simulink model "dec_2"  (R2013b)
settings: Solver=ode45  StartTime=0.0  StopTime=2500  RelTol=1e-3
undefined symbols (not defined in the file or in its folder): pfb_coeff_gen_calc, xlfda_numerator, xlipgetpartsetting
libraries: xbsIndex_r4 x1575, casper_library_delays x21, dspsigops x16, casper_library_misc x9, simulink x1, xps_library x1
(part 5 of 15)

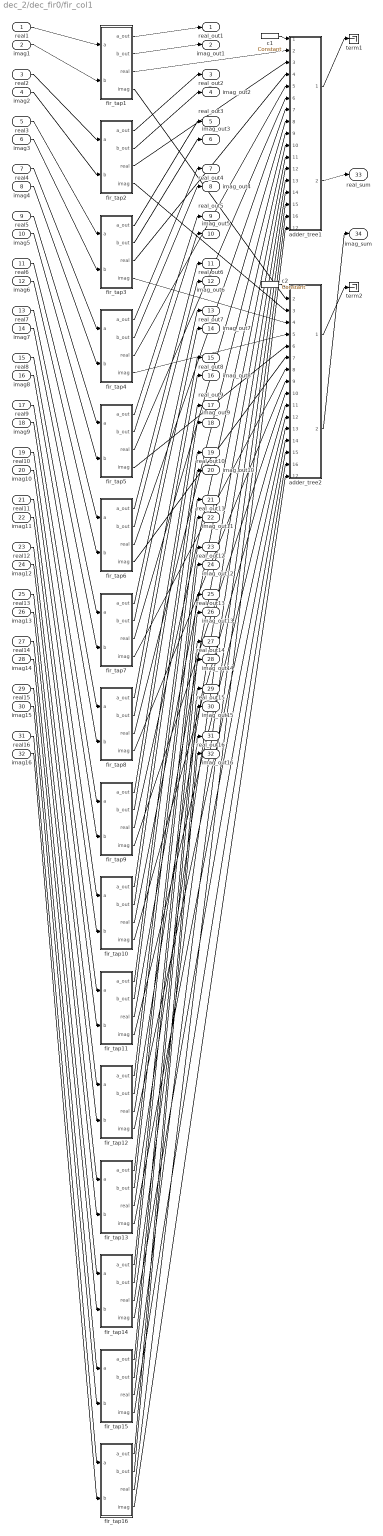
== system dec_2/dec_fir0/fir_col1 ==
  real1 : Inport
  imag1 : Inport  Port=2
  real2 : Inport  Port=3
  imag2 : Inport  Port=4
  real3 : Inport  Port=5
  imag3 : Inport  Port=6
  real4 : Inport  Port=7
  imag4 : Inport  Port=8
  real5 : Inport  Port=9
  imag5 : Inport  Port=10
  real6 : Inport  Port=11
  imag6 : Inport  Port=12
  real7 : Inport  Port=13
  imag7 : Inport  Port=14
  real8 : Inport  Port=15
  imag8 : Inport  Port=16
  real9 : Inport  Port=17
  imag9 : Inport  Port=18
  real10 : Inport  Port=19
  imag10 : Inport  Port=20
  real11 : Inport  Port=21
  imag11 : Inport  Port=22
  real12 : Inport  Port=23
  imag12 : Inport  Port=24
  real13 : Inport  Port=25
  imag13 : Inport  Port=26
  real14 : Inport  Port=27
  imag14 : Inport  Port=28
  real15 : Inport  Port=29
  imag15 : Inport  Port=30
  real16 : Inport  Port=31
  imag16 : Inport  Port=32
  adder_tree1 : Subsystem  AncestorBlock=casper_library_misc/adder_tree  mask(adder_tree){n_inputs=16, latency=1, adder_imp=DSP48, first_stage_hdl=on}
      mask prompts: n_inputs "Number of Inputs"; latency "Add Latency"; adder_imp "Adder implementation"; first_stage_hdl "Use behavioural HDL for first stage of adders"
      mask help:
      | Sums all inputs using a tree of adds and delays.
      |
      | Number of inputs: The number of inputs to the block to be summed
      | Add latency: The number of clock cycles to perform one addition (affects timing)..
      | Adder implementation: choice of fabric or DSP48E core, or behavioral HDL
      | Use behavioural HDL for first stage of adders: Causes the first stage of adders to be absorbed into DSP blocks if multipliers precede them (Virtex 5). Overrides Adder implementation
      mask init:
      | adder_tree_init(gcb, ...
      |     'n_inputs', n_inputs, ...
      |     'latency', latency, ...
      |     'adder_imp', adder_imp, ...
      |     'first_stage_hdl', first_stage_hdl);
      settings: AttributesFormatString=latency 4
      mask Help: eval('xlWeb(''http://casper.berkeley.edu/wiki/Adder_tree'')')
      mask TypeOptions adder_imp: Behavioral | Fabric | DSP48
  adder_tree2 : Subsystem  AncestorBlock=casper_library_misc/adder_tree  mask(adder_tree){n_inputs=16, latency=1, adder_imp=DSP48, first_stage_hdl=on}
      mask prompts: n_inputs "Number of Inputs"; latency "Add Latency"; adder_imp "Adder implementation"; first_stage_hdl "Use behavioural HDL for first stage of adders"
      mask help:
      | Sums all inputs using a tree of adds and delays.
      |
      | Number of inputs: The number of inputs to the block to be summed
      | Add latency: The number of clock cycles to perform one addition (affects timing)..
      | Adder implementation: choice of fabric or DSP48E core, or behavioral HDL
      | Use behavioural HDL for first stage of adders: Causes the first stage of adders to be absorbed into DSP blocks if multipliers precede them (Virtex 5). Overrides Adder implementation
      mask init:
      | adder_tree_init(gcb, ...
      |     'n_inputs', n_inputs, ...
      |     'latency', latency, ...
      |     'adder_imp', adder_imp, ...
      |     'first_stage_hdl', first_stage_hdl);
      settings: AttributesFormatString=latency 4
      mask Help: eval('xlWeb(''http://casper.berkeley.edu/wiki/Adder_tree'')')
      mask TypeOptions adder_imp: Behavioral | Fabric | DSP48
  c1 : xbsIndex_r4/Constant  const=1  gui_display_data_type=Fixed-point  arith_type=Signed (2's comp)  n_bits=16  bin_pt=14  preci_type=Single  exp_width=8  frac_width=24  explicit_period=on  period=1  equ=P=C  opselect=C  inp2=PCIN>>17  opr=+  inp1=P  carry=CIN  dbl_ovrd=off  block_type=constant
  c2 : xbsIndex_r4/Constant  const=1  gui_display_data_type=Fixed-point  arith_type=Signed (2's comp)  n_bits=16  bin_pt=14  preci_type=Single  exp_width=8  frac_width=24  explicit_period=on  period=1  equ=P=C  opselect=C  inp2=PCIN>>17  opr=+  inp1=P  carry=CIN  dbl_ovrd=off  block_type=constant
  fir_tap1 : Subsystem  AncestorBlock=casper_library_downconverter/fir_tap  mask(fir_tap){factor=0.0062127, latency=2, coeff_bit_width=25, coeff_bin_pt=24}
      mask prompts: latency "Mult latency"; coeff_bit_width "Coefficient bit width"; coeff_bin_pt "Coefficient binary point"
      mask help: Multiplies input data with factor specified.
      mask init:
      | fir_tap_init(gcb, ...
      |     'factor', factor, ...
      |     'latency', latency, ...
      |     'coeff_bit_width', coeff_bit_width, ...
      |     'coeff_bin_pt', coeff_bin_pt);
      mask Help: eval('xlWeb(''http://casper.berkeley.edu/wiki/Fir_tap'')')
  fir_tap10 : Subsystem  AncestorBlock=casper_library_downconverter/fir_tap  mask(fir_tap){factor=-0.0033818, latency=2, coeff_bit_width=25, coeff_bin_pt=24}
      mask prompts: latency "Mult latency"; coeff_bit_width "Coefficient bit width"; coeff_bin_pt "Coefficient binary point"
      mask help: Multiplies input data with factor specified.
      mask init:
      | fir_tap_init(gcb, ...
      |     'factor', factor, ...
      |     'latency', latency, ...
      |     'coeff_bit_width', coeff_bit_width, ...
      |     'coeff_bin_pt', coeff_bin_pt);
      mask Help: eval('xlWeb(''http://casper.berkeley.edu/wiki/Fir_tap'')')
  fir_tap11 : Subsystem  AncestorBlock=casper_library_downconverter/fir_tap  mask(fir_tap){factor=-0.0039996, latency=2, coeff_bit_width=25, coeff_bin_pt=24}
      mask prompts: latency "Mult latency"; coeff_bit_width "Coefficient bit width"; coeff_bin_pt "Coefficient binary point"
      mask help: Multiplies input data with factor specified.
      mask init:
      | fir_tap_init(gcb, ...
      |     'factor', factor, ...
      |     'latency', latency, ...
      |     'coeff_bit_width', coeff_bit_width, ...
      |     'coeff_bin_pt', coeff_bin_pt);
      mask Help: eval('xlWeb(''http://casper.berkeley.edu/wiki/Fir_tap'')')
  fir_tap12 : Subsystem  AncestorBlock=casper_library_downconverter/fir_tap  mask(fir_tap){factor=-0.0044174, latency=2, coeff_bit_width=25, coeff_bin_pt=24}
      mask prompts: latency "Mult latency"; coeff_bit_width "Coefficient bit width"; coeff_bin_pt "Coefficient binary point"
      mask help: Multiplies input data with factor specified.
      mask init:
      | fir_tap_init(gcb, ...
      |     'factor', factor, ...
      |     'latency', latency, ...
      |     'coeff_bit_width', coeff_bit_width, ...
      |     'coeff_bin_pt', coeff_bin_pt);
      mask Help: eval('xlWeb(''http://casper.berkeley.edu/wiki/Fir_tap'')')
  fir_tap13 : Subsystem  AncestorBlock=casper_library_downconverter/fir_tap  mask(fir_tap){factor=-0.0046295, latency=2, coeff_bit_width=25, coeff_bin_pt=24}
      mask prompts: latency "Mult latency"; coeff_bit_width "Coefficient bit width"; coeff_bin_pt "Coefficient binary point"
      mask help: Multiplies input data with factor specified.
      mask init:
      | fir_tap_init(gcb, ...
      |     'factor', factor, ...
      |     'latency', latency, ...
      |     'coeff_bit_width', coeff_bit_width, ...
      |     'coeff_bin_pt', coeff_bin_pt);
      mask Help: eval('xlWeb(''http://casper.berkeley.edu/wiki/Fir_tap'')')
  fir_tap14 : Subsystem  AncestorBlock=casper_library_downconverter/fir_tap  mask(fir_tap){factor=-0.0046386, latency=2, coeff_bit_width=25, coeff_bin_pt=24}
      mask prompts: latency "Mult latency"; coeff_bit_width "Coefficient bit width"; coeff_bin_pt "Coefficient binary point"
      mask help: Multiplies input data with factor specified.
      mask init:
      | fir_tap_init(gcb, ...
      |     'factor', factor, ...
      |     'latency', latency, ...
      |     'coeff_bit_width', coeff_bit_width, ...
      |     'coeff_bin_pt', coeff_bin_pt);
      mask Help: eval('xlWeb(''http://casper.berkeley.edu/wiki/Fir_tap'')')
  fir_tap15 : Subsystem  AncestorBlock=casper_library_downconverter/fir_tap  mask(fir_tap){factor=-0.0044554, latency=2, coeff_bit_width=25, coeff_bin_pt=24}
      mask prompts: latency "Mult latency"; coeff_bit_width "Coefficient bit width"; coeff_bin_pt "Coefficient binary point"
      mask help: Multiplies input data with factor specified.
      mask init:
      | fir_tap_init(gcb, ...
      |     'factor', factor, ...
      |     'latency', latency, ...
      |     'coeff_bit_width', coeff_bit_width, ...
      |     'coeff_bin_pt', coeff_bin_pt);
      mask Help: eval('xlWeb(''http://casper.berkeley.edu/wiki/Fir_tap'')')
  fir_tap16 : Subsystem  AncestorBlock=casper_library_downconverter/fir_tap  mask(fir_tap){factor=-0.0040983, latency=2, coeff_bit_width=25, coeff_bin_pt=24}
      mask prompts: latency "Mult latency"; coeff_bit_width "Coefficient bit width"; coeff_bin_pt "Coefficient binary point"
      mask help: Multiplies input data with factor specified.
      mask init:
      | fir_tap_init(gcb, ...
      |     'factor', factor, ...
      |     'latency', latency, ...
      |     'coeff_bit_width', coeff_bit_width, ...
      |     'coeff_bin_pt', coeff_bin_pt);
      mask Help: eval('xlWeb(''http://casper.berkeley.edu/wiki/Fir_tap'')')
  fir_tap2 : Subsystem  AncestorBlock=casper_library_downconverter/fir_tap  mask(fir_tap){factor=0.0053266, latency=2, coeff_bit_width=25, coeff_bin_pt=24}
      mask prompts: latency "Mult latency"; coeff_bit_width "Coefficient bit width"; coeff_bin_pt "Coefficient binary point"
      mask help: Multiplies input data with factor specified.
      mask init:
      | fir_tap_init(gcb, ...
      |     'factor', factor, ...
      |     'latency', latency, ...
      |     'coeff_bit_width', coeff_bit_width, ...
      |     'coeff_bin_pt', coeff_bin_pt);
      mask Help: eval('xlWeb(''http://casper.berkeley.edu/wiki/Fir_tap'')')
  fir_tap3 : Subsystem  AncestorBlock=casper_library_downconverter/fir_tap  mask(fir_tap){factor=0.0042757, latency=2, coeff_bit_width=25, coeff_bin_pt=24}
      mask prompts: latency "Mult latency"; coeff_bit_width "Coefficient bit width"; coeff_bin_pt "Coefficient binary point"
      mask help: Multiplies input data with factor specified.
      mask init:
      | fir_tap_init(gcb, ...
      |     'factor', factor, ...
      |     'latency', latency, ...
      |     'coeff_bit_width', coeff_bit_width, ...
      |     'coeff_bin_pt', coeff_bin_pt);
      mask Help: eval('xlWeb(''http://casper.berkeley.edu/wiki/Fir_tap'')')
  fir_tap4 : Subsystem  AncestorBlock=casper_library_downconverter/fir_tap  mask(fir_tap){factor=0.0031122, latency=2, coeff_bit_width=25, coeff_bin_pt=24}
      mask prompts: latency "Mult latency"; coeff_bit_width "Coefficient bit width"; coeff_bin_pt "Coefficient binary point"
      mask help: Multiplies input data with factor specified.
      mask init:
      | fir_tap_init(gcb, ...
      |     'factor', factor, ...
      |     'latency', latency, ...
      |     'coeff_bit_width', coeff_bit_width, ...
      |     'coeff_bin_pt', coeff_bin_pt);
      mask Help: eval('xlWeb(''http://casper.berkeley.edu/wiki/Fir_tap'')')
  fir_tap5 : Subsystem  AncestorBlock=casper_library_downconverter/fir_tap  mask(fir_tap){factor=0.00189, latency=2, coeff_bit_width=25, coeff_bin_pt=24}
      mask prompts: latency "Mult latency"; coeff_bit_width "Coefficient bit width"; coeff_bin_pt "Coefficient binary point"
      mask help: Multiplies input data with factor specified.
      mask init:
      | fir_tap_init(gcb, ...
      |     'factor', factor, ...
      |     'latency', latency, ...
      |     'coeff_bit_width', coeff_bit_width, ...
      |     'coeff_bin_pt', coeff_bin_pt);
      mask Help: eval('xlWeb(''http://casper.berkeley.edu/wiki/Fir_tap'')')
  fir_tap6 : Subsystem  AncestorBlock=casper_library_downconverter/fir_tap  mask(fir_tap){factor=0.00066203, latency=2, coeff_bit_width=25, coeff_bin_pt=24}
      mask prompts: latency "Mult latency"; coeff_bit_width "Coefficient bit width"; coeff_bin_pt "Coefficient binary point"
      mask help: Multiplies input data with factor specified.
      mask init:
      | fir_tap_init(gcb, ...
      |     'factor', factor, ...
      |     'latency', latency, ...
      |     'coeff_bit_width', coeff_bit_width, ...
      |     'coeff_bin_pt', coeff_bin_pt);
      mask Help: eval('xlWeb(''http://casper.berkeley.edu/wiki/Fir_tap'')')
  fir_tap7 : Subsystem  AncestorBlock=casper_library_downconverter/fir_tap  mask(fir_tap){factor=-0.00052147, latency=2, coeff_bit_width=25, coeff_bin_pt=24}
      mask prompts: latency "Mult latency"; coeff_bit_width "Coefficient bit width"; coeff_bin_pt "Coefficient binary point"
      mask help: Multiplies input data with factor specified.
      mask init:
      | fir_tap_init(gcb, ...
      |     'factor', factor, ...
      |     'latency', latency, ...
      |     'coeff_bit_width', coeff_bit_width, ...
      |     'coeff_bin_pt', coeff_bin_pt);
      mask Help: eval('xlWeb(''http://casper.berkeley.edu/wiki/Fir_tap'')')
  fir_tap8 : Subsystem  AncestorBlock=casper_library_downconverter/fir_tap  mask(fir_tap){factor=-0.001615, latency=2, coeff_bit_width=25, coeff_bin_pt=24}
      mask prompts: latency "Mult latency"; coeff_bit_width "Coefficient bit width"; coeff_bin_pt "Coefficient binary point"
      mask help: Multiplies input data with factor specified.
      mask init:
      | fir_tap_init(gcb, ...
      |     'factor', factor, ...
      |     'latency', latency, ...
      |     'coeff_bit_width', coeff_bit_width, ...
      |     'coeff_bin_pt', coeff_bin_pt);
      mask Help: eval('xlWeb(''http://casper.berkeley.edu/wiki/Fir_tap'')')
  fir_tap9 : Subsystem  AncestorBlock=casper_library_downconverter/fir_tap  mask(fir_tap){factor=-0.0025791, latency=2, coeff_bit_width=25, coeff_bin_pt=24}
      mask prompts: latency "Mult latency"; coeff_bit_width "Coefficient bit width"; coeff_bin_pt "Coefficient binary point"
      mask help: Multiplies input data with factor specified.
      mask init:
      | fir_tap_init(gcb, ...
      |     'factor', factor, ...
      |     'latency', latency, ...
      |     'coeff_bit_width', coeff_bit_width, ...
      |     'coeff_bin_pt', coeff_bin_pt);
      mask Help: eval('xlWeb(''http://casper.berkeley.edu/wiki/Fir_tap'')')
  term1 : Terminator
  term2 : Terminator
  real_out1 : Outport
  imag_out1 : Outport  Port=2
  real_out2 : Outport  Port=3
  imag_out2 : Outport  Port=4
  real_out3 : Outport  Port=5
  imag_out3 : Outport  Port=6
  real_out4 : Outport  Port=7
  imag_out4 : Outport  Port=8
  real_out5 : Outport  Port=9
  imag_out5 : Outport  Port=10
  real_out6 : Outport  Port=11
  imag_out6 : Outport  Port=12
  real_out7 : Outport  Port=13
  imag_out7 : Outport  Port=14
  real_out8 : Outport  Port=15
  imag_out8 : Outport  Port=16
  real_out9 : Outport  Port=17
  imag_out9 : Outport  Port=18
  real_out10 : Outport  Port=19
  imag_out10 : Outport  Port=20
  real_out11 : Outport  Port=21
  imag_out11 : Outport  Port=22
  real_out12 : Outport  Port=23
  imag_out12 : Outport  Port=24
  real_out13 : Outport  Port=25
  imag_out13 : Outport  Port=26
  real_out14 : Outport  Port=27
  imag_out14 : Outport  Port=28
  real_out15 : Outport  Port=29
  imag_out15 : Outport  Port=30
  real_out16 : Outport  Port=31
  imag_out16 : Outport  Port=32
  real_sum : Outport  Port=33
  imag_sum : Outport  Port=34
  wires:
  adder_tree1/1(sync_out) -> term1/1
  adder_tree2/1(sync_out) -> term2/1
  c1/1 -> adder_tree1/1(sync)
  c2/1 -> adder_tree2/1(sync)
  adder_tree1/2(dout) -> real_sum/1
  adder_tree2/2(dout) -> imag_sum/1
  real1/1 -> fir_tap1/1(a)
  imag1/1 -> fir_tap1/2(b)
  fir_tap1/1(a_out) -> real_out1/1
  fir_tap1/2(b_out) -> imag_out1/1
  fir_tap1/3(real) -> adder_tree1/2(din1)
  fir_tap1/4(imag) -> adder_tree2/2(din1)
  real2/1 -> fir_tap2/1(a)
  imag2/1 -> fir_tap2/2(b)
  fir_tap2/1(a_out) -> real_out2/1
  fir_tap2/2(b_out) -> imag_out2/1
  fir_tap2/3(real) -> adder_tree1/3(din2)
  fir_tap2/4(imag) -> adder_tree2/3(din2)
  real3/1 -> fir_tap3/1(a)
  imag3/1 -> fir_tap3/2(b)
  fir_tap3/1(a_out) -> real_out3/1
  fir_tap3/2(b_out) -> imag_out3/1
  fir_tap3/3(real) -> adder_tree1/4(din3)
  fir_tap3/4(imag) -> adder_tree2/4(din3)
  real4/1 -> fir_tap4/1(a)
  imag4/1 -> fir_tap4/2(b)
  fir_tap4/1(a_out) -> real_out4/1
  fir_tap4/2(b_out) -> imag_out4/1
  fir_tap4/3(real) -> adder_tree1/5(din4)
  fir_tap4/4(imag) -> adder_tree2/5(din4)
  real5/1 -> fir_tap5/1(a)
  imag5/1 -> fir_tap5/2(b)
  fir_tap5/1(a_out) -> real_out5/1
  fir_tap5/2(b_out) -> imag_out5/1
  fir_tap5/3(real) -> adder_tree1/6(din5)
  fir_tap5/4(imag) -> adder_tree2/6(din5)
  real6/1 -> fir_tap6/1(a)
  imag6/1 -> fir_tap6/2(b)
  fir_tap6/1(a_out) -> real_out6/1
  fir_tap6/2(b_out) -> imag_out6/1
  fir_tap6/3(real) -> adder_tree1/7(din6)
  fir_tap6/4(imag) -> adder_tree2/7(din6)
  real7/1 -> fir_tap7/1(a)
  imag7/1 -> fir_tap7/2(b)
  fir_tap7/1(a_out) -> real_out7/1
  fir_tap7/2(b_out) -> imag_out7/1
  fir_tap7/3(real) -> adder_tree1/8(din7)
  fir_tap7/4(imag) -> adder_tree2/8(din7)
  real8/1 -> fir_tap8/1(a)
  imag8/1 -> fir_tap8/2(b)
  fir_tap8/1(a_out) -> real_out8/1
  fir_tap8/2(b_out) -> imag_out8/1
  fir_tap8/3(real) -> adder_tree1/9(din8)
  fir_tap8/4(imag) -> adder_tree2/9(din8)
  real9/1 -> fir_tap9/1(a)
  imag9/1 -> fir_tap9/2(b)
  fir_tap9/1(a_out) -> real_out9/1
  fir_tap9/2(b_out) -> imag_out9/1
  fir_tap9/3(real) -> adder_tree1/10(din9)
  fir_tap9/4(imag) -> adder_tree2/10(din9)
  real10/1 -> fir_tap10/1(a)
  imag10/1 -> fir_tap10/2(b)
  fir_tap10/1(a_out) -> real_out10/1
  fir_tap10/2(b_out) -> imag_out10/1
  fir_tap10/3(real) -> adder_tree1/11(din10)
  fir_tap10/4(imag) -> adder_tree2/11(din10)
  real11/1 -> fir_tap11/1(a)
  imag11/1 -> fir_tap11/2(b)
  fir_tap11/1(a_out) -> real_out11/1
  fir_tap11/2(b_out) -> imag_out11/1
  fir_tap11/3(real) -> adder_tree1/12(din11)
  fir_tap11/4(imag) -> adder_tree2/12(din11)
  real12/1 -> fir_tap12/1(a)
  imag12/1 -> fir_tap12/2(b)
  fir_tap12/1(a_out) -> real_out12/1
  fir_tap12/2(b_out) -> imag_out12/1
  fir_tap12/3(real) -> adder_tree1/13(din12)
  fir_tap12/4(imag) -> adder_tree2/13(din12)
  real13/1 -> fir_tap13/1(a)
  imag13/1 -> fir_tap13/2(b)
  fir_tap13/1(a_out) -> real_out13/1
  fir_tap13/2(b_out) -> imag_out13/1
  fir_tap13/3(real) -> adder_tree1/14(din13)
  fir_tap13/4(imag) -> adder_tree2/14(din13)
  real14/1 -> fir_tap14/1(a)
  imag14/1 -> fir_tap14/2(b)
  fir_tap14/1(a_out) -> real_out14/1
  fir_tap14/2(b_out) -> imag_out14/1
  fir_tap14/3(real) -> adder_tree1/15(din14)
  fir_tap14/4(imag) -> adder_tree2/15(din14)
  real15/1 -> fir_tap15/1(a)
  imag15/1 -> fir_tap15/2(b)
  fir_tap15/1(a_out) -> real_out15/1
  fir_tap15/2(b_out) -> imag_out15/1
  fir_tap15/3(real) -> adder_tree1/16(din15)
  fir_tap15/4(imag) -> adder_tree2/16(din15)
  real16/1 -> fir_tap16/1(a)
  imag16/1 -> fir_tap16/2(b)
  fir_tap16/1(a_out) -> real_out16/1
  fir_tap16/2(b_out) -> imag_out16/1
  fir_tap16/3(real) -> adder_tree1/17(din16)
  fir_tap16/4(imag) -> adder_tree2/17(din16)

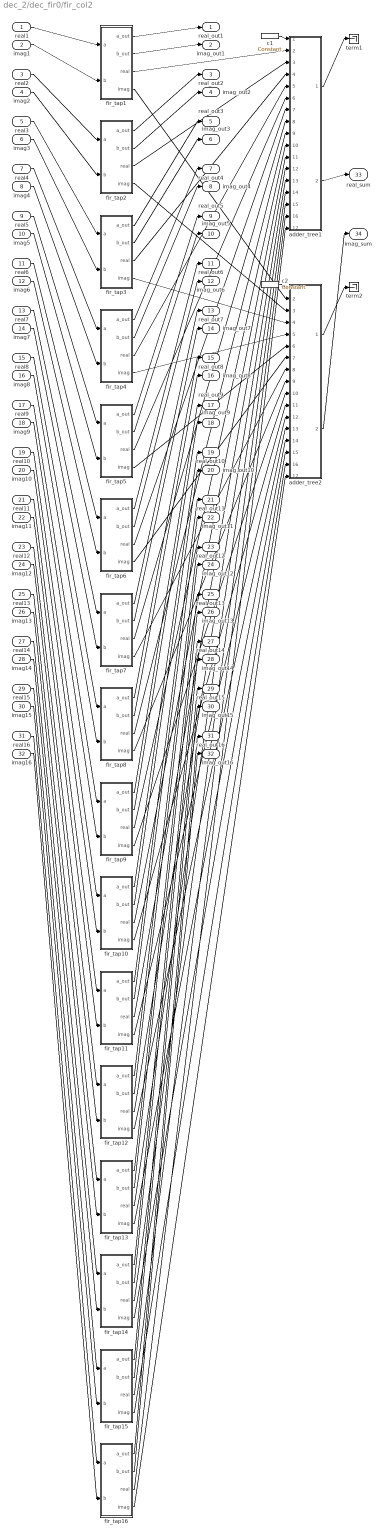
== system dec_2/dec_fir0/fir_col2 ==
  real1 : Inport
  imag1 : Inport  Port=2
  real2 : Inport  Port=3
  imag2 : Inport  Port=4
  real3 : Inport  Port=5
  imag3 : Inport  Port=6
  real4 : Inport  Port=7
  imag4 : Inport  Port=8
  real5 : Inport  Port=9
  imag5 : Inport  Port=10
  real6 : Inport  Port=11
  imag6 : Inport  Port=12
  real7 : Inport  Port=13
  imag7 : Inport  Port=14
  real8 : Inport  Port=15
  imag8 : Inport  Port=16
  real9 : Inport  Port=17
  imag9 : Inport  Port=18
  real10 : Inport  Port=19
  imag10 : Inport  Port=20
  real11 : Inport  Port=21
  imag11 : Inport  Port=22
  real12 : Inport  Port=23
  imag12 : Inport  Port=24
  real13 : Inport  Port=25
  imag13 : Inport  Port=26
  real14 : Inport  Port=27
  imag14 : Inport  Port=28
  real15 : Inport  Port=29
  imag15 : Inport  Port=30
  real16 : Inport  Port=31
  imag16 : Inport  Port=32
  adder_tree1 : Subsystem  AncestorBlock=casper_library_misc/adder_tree  mask(adder_tree){n_inputs=16, latency=1, adder_imp=DSP48, first_stage_hdl=on}
      mask prompts: n_inputs "Number of Inputs"; latency "Add Latency"; adder_imp "Adder implementation"; first_stage_hdl "Use behavioural HDL for first stage of adders"
      mask help:
      | Sums all inputs using a tree of adds and delays.
      |
      | Number of inputs: The number of inputs to the block to be summed
      | Add latency: The number of clock cycles to perform one addition (affects timing)..
      | Adder implementation: choice of fabric or DSP48E core, or behavioral HDL
      | Use behavioural HDL for first stage of adders: Causes the first stage of adders to be absorbed into DSP blocks if multipliers precede them (Virtex 5). Overrides Adder implementation
      mask init:
      | adder_tree_init(gcb, ...
      |     'n_inputs', n_inputs, ...
      |     'latency', latency, ...
      |     'adder_imp', adder_imp, ...
      |     'first_stage_hdl', first_stage_hdl);
      settings: AttributesFormatString=latency 4
      mask Help: eval('xlWeb(''http://casper.berkeley.edu/wiki/Adder_tree'')')
      mask TypeOptions adder_imp: Behavioral | Fabric | DSP48
  adder_tree2 : Subsystem  AncestorBlock=casper_library_misc/adder_tree  mask(adder_tree){n_inputs=16, latency=1, adder_imp=DSP48, first_stage_hdl=on}
      mask prompts: n_inputs "Number of Inputs"; latency "Add Latency"; adder_imp "Adder implementation"; first_stage_hdl "Use behavioural HDL for first stage of adders"
      mask help:
      | Sums all inputs using a tree of adds and delays.
      |
      | Number of inputs: The number of inputs to the block to be summed
      | Add latency: The number of clock cycles to perform one addition (affects timing)..
      | Adder implementation: choice of fabric or DSP48E core, or behavioral HDL
      | Use behavioural HDL for first stage of adders: Causes the first stage of adders to be absorbed into DSP blocks if multipliers precede them (Virtex 5). Overrides Adder implementation
      mask init:
      | adder_tree_init(gcb, ...
      |     'n_inputs', n_inputs, ...
      |     'latency', latency, ...
      |     'adder_imp', adder_imp, ...
      |     'first_stage_hdl', first_stage_hdl);
      settings: AttributesFormatString=latency 4
      mask Help: eval('xlWeb(''http://casper.berkeley.edu/wiki/Adder_tree'')')
      mask TypeOptions adder_imp: Behavioral | Fabric | DSP48
  c1 : xbsIndex_r4/Constant  const=1  gui_display_data_type=Fixed-point  arith_type=Signed (2's comp)  n_bits=16  bin_pt=14  preci_type=Single  exp_width=8  frac_width=24  explicit_period=on  period=1  equ=P=C  opselect=C  inp2=PCIN>>17  opr=+  inp1=P  carry=CIN  dbl_ovrd=off  block_type=constant
  c2 : xbsIndex_r4/Constant  const=1  gui_display_data_type=Fixed-point  arith_type=Signed (2's comp)  n_bits=16  bin_pt=14  preci_type=Single  exp_width=8  frac_width=24  explicit_period=on  period=1  equ=P=C  opselect=C  inp2=PCIN>>17  opr=+  inp1=P  carry=CIN  dbl_ovrd=off  block_type=constant
  fir_tap1 : Subsystem  AncestorBlock=casper_library_downconverter/fir_tap  mask(fir_tap){factor=-0.011813, latency=2, coeff_bit_width=25, coeff_bin_pt=24}
      mask prompts: latency "Mult latency"; coeff_bit_width "Coefficient bit width"; coeff_bin_pt "Coefficient binary point"
      mask help: Multiplies input data with factor specified.
      mask init:
      | fir_tap_init(gcb, ...
      |     'factor', factor, ...
      |     'latency', latency, ...
      |     'coeff_bit_width', coeff_bit_width, ...
      |     'coeff_bin_pt', coeff_bin_pt);
      mask Help: eval('xlWeb(''http://casper.berkeley.edu/wiki/Fir_tap'')')
  fir_tap10 : Subsystem  AncestorBlock=casper_library_downconverter/fir_tap  mask(fir_tap){factor=0.0046863, latency=2, coeff_bit_width=25, coeff_bin_pt=24}
      mask prompts: latency "Mult latency"; coeff_bit_width "Coefficient bit width"; coeff_bin_pt "Coefficient binary point"
      mask help: Multiplies input data with factor specified.
      mask init:
      | fir_tap_init(gcb, ...
      |     'factor', factor, ...
      |     'latency', latency, ...
      |     'coeff_bit_width', coeff_bit_width, ...
      |     'coeff_bin_pt', coeff_bin_pt);
      mask Help: eval('xlWeb(''http://casper.berkeley.edu/wiki/Fir_tap'')')
  fir_tap11 : Subsystem  AncestorBlock=casper_library_downconverter/fir_tap  mask(fir_tap){factor=0.005858, latency=2, coeff_bit_width=25, coeff_bin_pt=24}
      mask prompts: latency "Mult latency"; coeff_bit_width "Coefficient bit width"; coeff_bin_pt "Coefficient binary point"
      mask help: Multiplies input data with factor specified.
      mask init:
      | fir_tap_init(gcb, ...
      |     'factor', factor, ...
      |     'latency', latency, ...
      |     'coeff_bit_width', coeff_bit_width, ...
      |     'coeff_bin_pt', coeff_bin_pt);
      mask Help: eval('xlWeb(''http://casper.berkeley.edu/wiki/Fir_tap'')')
  fir_tap12 : Subsystem  AncestorBlock=casper_library_downconverter/fir_tap  mask(fir_tap){factor=0.0067112, latency=2, coeff_bit_width=25, coeff_bin_pt=24}
      mask prompts: latency "Mult latency"; coeff_bit_width "Coefficient bit width"; coeff_bin_pt "Coefficient binary point"
      mask help: Multiplies input data with factor specified.
      mask init:
      | fir_tap_init(gcb, ...
      |     'factor', factor, ...
      |     'latency', latency, ...
      |     'coeff_bit_width', coeff_bit_width, ...
      |     'coeff_bin_pt', coeff_bin_pt);
      mask Help: eval('xlWeb(''http://casper.berkeley.edu/wiki/Fir_tap'')')
  fir_tap13 : Subsystem  AncestorBlock=casper_library_downconverter/fir_tap  mask(fir_tap){factor=0.0072334, latency=2, coeff_bit_width=25, coeff_bin_pt=24}
      mask prompts: latency "Mult latency"; coeff_bit_width "Coefficient bit width"; coeff_bin_pt "Coefficient binary point"
      mask help: Multiplies input data with factor specified.
      mask init:
      | fir_tap_init(gcb, ...
      |     'factor', factor, ...
      |     'latency', latency, ...
      |     'coeff_bit_width', coeff_bit_width, ...
      |     'coeff_bin_pt', coeff_bin_pt);
      mask Help: eval('xlWeb(''http://casper.berkeley.edu/wiki/Fir_tap'')')
  fir_tap14 : Subsystem  AncestorBlock=casper_library_downconverter/fir_tap  mask(fir_tap){factor=0.0074255, latency=2, coeff_bit_width=25, coeff_bin_pt=24}
      mask prompts: latency "Mult latency"; coeff_bit_width "Coefficient bit width"; coeff_bin_pt "Coefficient binary point"
      mask help: Multiplies input data with factor specified.
      mask init:
      | fir_tap_init(gcb, ...
      |     'factor', factor, ...
      |     'latency', latency, ...
      |     'coeff_bit_width', coeff_bit_width, ...
      |     'coeff_bin_pt', coeff_bin_pt);
      mask Help: eval('xlWeb(''http://casper.berkeley.edu/wiki/Fir_tap'')')
  fir_tap15 : Subsystem  AncestorBlock=casper_library_downconverter/fir_tap  mask(fir_tap){factor=0.007301, latency=2, coeff_bit_width=25, coeff_bin_pt=24}
      mask prompts: latency "Mult latency"; coeff_bit_width "Coefficient bit width"; coeff_bin_pt "Coefficient binary point"
      mask help: Multiplies input data with factor specified.
      mask init:
      | fir_tap_init(gcb, ...
      |     'factor', factor, ...
      |     'latency', latency, ...
      |     'coeff_bit_width', coeff_bit_width, ...
      |     'coeff_bin_pt', coeff_bin_pt);
      mask Help: eval('xlWeb(''http://casper.berkeley.edu/wiki/Fir_tap'')')
  fir_tap16 : Subsystem  AncestorBlock=casper_library_downconverter/fir_tap  mask(fir_tap){factor=0.0068851, latency=2, coeff_bit_width=25, coeff_bin_pt=24}
      mask prompts: latency "Mult latency"; coeff_bit_width "Coefficient bit width"; coeff_bin_pt "Coefficient binary point"
      mask help: Multiplies input data with factor specified.
      mask init:
      | fir_tap_init(gcb, ...
      |     'factor', factor, ...
      |     'latency', latency, ...
      |     'coeff_bit_width', coeff_bit_width, ...
      |     'coeff_bin_pt', coeff_bin_pt);
      mask Help: eval('xlWeb(''http://casper.berkeley.edu/wiki/Fir_tap'')')
  fir_tap2 : Subsystem  AncestorBlock=casper_library_downconverter/fir_tap  mask(fir_tap){factor=-0.010354, latency=2, coeff_bit_width=25, coeff_bin_pt=24}
      mask prompts: latency "Mult latency"; coeff_bit_width "Coefficient bit width"; coeff_bin_pt "Coefficient binary point"
      mask help: Multiplies input data with factor specified.
      mask init:
      | fir_tap_init(gcb, ...
      |     'factor', factor, ...
      |     'latency', latency, ...
      |     'coeff_bit_width', coeff_bit_width, ...
      |     'coeff_bin_pt', coeff_bin_pt);
      mask Help: eval('xlWeb(''http://casper.berkeley.edu/wiki/Fir_tap'')')
  fir_tap3 : Subsystem  AncestorBlock=casper_library_downconverter/fir_tap  mask(fir_tap){factor=-0.0085971, latency=2, coeff_bit_width=25, coeff_bin_pt=24}
      mask prompts: latency "Mult latency"; coeff_bit_width "Coefficient bit width"; coeff_bin_pt "Coefficient binary point"
      mask help: Multiplies input data with factor specified.
      mask init:
      | fir_tap_init(gcb, ...
      |     'factor', factor, ...
      |     'latency', latency, ...
      |     'coeff_bit_width', coeff_bit_width, ...
      |     'coeff_bin_pt', coeff_bin_pt);
      mask Help: eval('xlWeb(''http://casper.berkeley.edu/wiki/Fir_tap'')')
  fir_tap4 : Subsystem  AncestorBlock=casper_library_downconverter/fir_tap  mask(fir_tap){factor=-0.0066339, latency=2, coeff_bit_width=25, coeff_bin_pt=24}
      mask prompts: latency "Mult latency"; coeff_bit_width "Coefficient bit width"; coeff_bin_pt "Coefficient binary point"
      mask help: Multiplies input data with factor specified.
      mask init:
      | fir_tap_init(gcb, ...
      |     'factor', factor, ...
      |     'latency', latency, ...
      |     'coeff_bit_width', coeff_bit_width, ...
      |     'coeff_bin_pt', coeff_bin_pt);
      mask Help: eval('xlWeb(''http://casper.berkeley.edu/wiki/Fir_tap'')')
  fir_tap5 : Subsystem  AncestorBlock=casper_library_downconverter/fir_tap  mask(fir_tap){factor=-0.0045559, latency=2, coeff_bit_width=25, coeff_bin_pt=24}
      mask prompts: latency "Mult latency"; coeff_bit_width "Coefficient bit width"; coeff_bin_pt "Coefficient binary point"
      mask help: Multiplies input data with factor specified.
      mask init:
      | fir_tap_init(gcb, ...
      |     'factor', factor, ...
      |     'latency', latency, ...
      |     'coeff_bit_width', coeff_bit_width, ...
      |     'coeff_bin_pt', coeff_bin_pt);
      mask Help: eval('xlWeb(''http://casper.berkeley.edu/wiki/Fir_tap'')')
  fir_tap6 : Subsystem  AncestorBlock=casper_library_downconverter/fir_tap  mask(fir_tap){factor=-0.002452, latency=2, coeff_bit_width=25, coeff_bin_pt=24}
      mask prompts: latency "Mult latency"; coeff_bit_width "Coefficient bit width"; coeff_bin_pt "Coefficient binary point"
      mask help: Multiplies input data with factor specified.
      mask init:
      | fir_tap_init(gcb, ...
      |     'factor', factor, ...
      |     'latency', latency, ...
      |     'coeff_bit_width', coeff_bit_width, ...
      |     'coeff_bin_pt', coeff_bin_pt);
      mask Help: eval('xlWeb(''http://casper.berkeley.edu/wiki/Fir_tap'')')
  fir_tap7 : Subsystem  AncestorBlock=casper_library_downconverter/fir_tap  mask(fir_tap){factor=-0.00040564, latency=2, coeff_bit_width=25, coeff_bin_pt=24}
      mask prompts: latency "Mult latency"; coeff_bit_width "Coefficient bit width"; coeff_bin_pt "Coefficient binary point"
      mask help: Multiplies input data with factor specified.
      mask init:
      | fir_tap_init(gcb, ...
      |     'factor', factor, ...
      |     'latency', latency, ...
      |     'coeff_bit_width', coeff_bit_width, ...
      |     'coeff_bin_pt', coeff_bin_pt);
      mask Help: eval('xlWeb(''http://casper.berkeley.edu/wiki/Fir_tap'')')
  fir_tap8 : Subsystem  AncestorBlock=casper_library_downconverter/fir_tap  mask(fir_tap){factor=0.0015077, latency=2, coeff_bit_width=25, coeff_bin_pt=24}
      mask prompts: latency "Mult latency"; coeff_bit_width "Coefficient bit width"; coeff_bin_pt "Coefficient binary point"
      mask help: Multiplies input data with factor specified.
      mask init:
      | fir_tap_init(gcb, ...
      |     'factor', factor, ...
      |     'latency', latency, ...
      |     'coeff_bit_width', coeff_bit_width, ...
      |     'coeff_bin_pt', coeff_bin_pt);
      mask Help: eval('xlWeb(''http://casper.berkeley.edu/wiki/Fir_tap'')')
  fir_tap9 : Subsystem  AncestorBlock=casper_library_downconverter/fir_tap  mask(fir_tap){factor=0.0032228, latency=2, coeff_bit_width=25, coeff_bin_pt=24}
      mask prompts: latency "Mult latency"; coeff_bit_width "Coefficient bit width"; coeff_bin_pt "Coefficient binary point"
      mask help: Multiplies input data with factor specified.
      mask init:
      | fir_tap_init(gcb, ...
      |     'factor', factor, ...
      |     'latency', latency, ...
      |     'coeff_bit_width', coeff_bit_width, ...
      |     'coeff_bin_pt', coeff_bin_pt);
      mask Help: eval('xlWeb(''http://casper.berkeley.edu/wiki/Fir_tap'')')
  term1 : Terminator
  term2 : Terminator
  real_out1 : Outport
  imag_out1 : Outport  Port=2
  real_out2 : Outport  Port=3
  imag_out2 : Outport  Port=4
  real_out3 : Outport  Port=5
  imag_out3 : Outport  Port=6
  real_out4 : Outport  Port=7
  imag_out4 : Outport  Port=8
  real_out5 : Outport  Port=9
  imag_out5 : Outport  Port=10
  real_out6 : Outport  Port=11
  imag_out6 : Outport  Port=12
  real_out7 : Outport  Port=13
  imag_out7 : Outport  Port=14
  real_out8 : Outport  Port=15
  imag_out8 : Outport  Port=16
  real_out9 : Outport  Port=17
  imag_out9 : Outport  Port=18
  real_out10 : Outport  Port=19
  imag_out10 : Outport  Port=20
  real_out11 : Outport  Port=21
  imag_out11 : Outport  Port=22
  real_out12 : Outport  Port=23
  imag_out12 : Outport  Port=24
  real_out13 : Outport  Port=25
  imag_out13 : Outport  Port=26
  real_out14 : Outport  Port=27
  imag_out14 : Outport  Port=28
  real_out15 : Outport  Port=29
  imag_out15 : Outport  Port=30
  real_out16 : Outport  Port=31
  imag_out16 : Outport  Port=32
  real_sum : Outport  Port=33
  imag_sum : Outport  Port=34
  wires:
  adder_tree1/1(sync_out) -> term1/1
  adder_tree2/1(sync_out) -> term2/1
  c1/1 -> adder_tree1/1(sync)
  c2/1 -> adder_tree2/1(sync)
  adder_tree1/2(dout) -> real_sum/1
  adder_tree2/2(dout) -> imag_sum/1
  real1/1 -> fir_tap1/1(a)
  imag1/1 -> fir_tap1/2(b)
  fir_tap1/1(a_out) -> real_out1/1
  fir_tap1/2(b_out) -> imag_out1/1
  fir_tap1/3(real) -> adder_tree1/2(din1)
  fir_tap1/4(imag) -> adder_tree2/2(din1)
  real2/1 -> fir_tap2/1(a)
  imag2/1 -> fir_tap2/2(b)
  fir_tap2/1(a_out) -> real_out2/1
  fir_tap2/2(b_out) -> imag_out2/1
  fir_tap2/3(real) -> adder_tree1/3(din2)
  fir_tap2/4(imag) -> adder_tree2/3(din2)
  real3/1 -> fir_tap3/1(a)
  imag3/1 -> fir_tap3/2(b)
  fir_tap3/1(a_out) -> real_out3/1
  fir_tap3/2(b_out) -> imag_out3/1
  fir_tap3/3(real) -> adder_tree1/4(din3)
  fir_tap3/4(imag) -> adder_tree2/4(din3)
  real4/1 -> fir_tap4/1(a)
  imag4/1 -> fir_tap4/2(b)
  fir_tap4/1(a_out) -> real_out4/1
  fir_tap4/2(b_out) -> imag_out4/1
  fir_tap4/3(real) -> adder_tree1/5(din4)
  fir_tap4/4(imag) -> adder_tree2/5(din4)
  real5/1 -> fir_tap5/1(a)
  imag5/1 -> fir_tap5/2(b)
  fir_tap5/1(a_out) -> real_out5/1
  fir_tap5/2(b_out) -> imag_out5/1
  fir_tap5/3(real) -> adder_tree1/6(din5)
  fir_tap5/4(imag) -> adder_tree2/6(din5)
  real6/1 -> fir_tap6/1(a)
  imag6/1 -> fir_tap6/2(b)
  fir_tap6/1(a_out) -> real_out6/1
  fir_tap6/2(b_out) -> imag_out6/1
  fir_tap6/3(real) -> adder_tree1/7(din6)
  fir_tap6/4(imag) -> adder_tree2/7(din6)
  real7/1 -> fir_tap7/1(a)
  imag7/1 -> fir_tap7/2(b)
  fir_tap7/1(a_out) -> real_out7/1
  fir_tap7/2(b_out) -> imag_out7/1
  fir_tap7/3(real) -> adder_tree1/8(din7)
  fir_tap7/4(imag) -> adder_tree2/8(din7)
  real8/1 -> fir_tap8/1(a)
  imag8/1 -> fir_tap8/2(b)
  fir_tap8/1(a_out) -> real_out8/1
  fir_tap8/2(b_out) -> imag_out8/1
  fir_tap8/3(real) -> adder_tree1/9(din8)
  fir_tap8/4(imag) -> adder_tree2/9(din8)
  real9/1 -> fir_tap9/1(a)
  imag9/1 -> fir_tap9/2(b)
  fir_tap9/1(a_out) -> real_out9/1
  fir_tap9/2(b_out) -> imag_out9/1
  fir_tap9/3(real) -> adder_tree1/10(din9)
  fir_tap9/4(imag) -> adder_tree2/10(din9)
  real10/1 -> fir_tap10/1(a)
  imag10/1 -> fir_tap10/2(b)
  fir_tap10/1(a_out) -> real_out10/1
  fir_tap10/2(b_out) -> imag_out10/1
  fir_tap10/3(real) -> adder_tree1/11(din10)
  fir_tap10/4(imag) -> adder_tree2/11(din10)
  real11/1 -> fir_tap11/1(a)
  imag11/1 -> fir_tap11/2(b)
  fir_tap11/1(a_out) -> real_out11/1
  fir_tap11/2(b_out) -> imag_out11/1
  fir_tap11/3(real) -> adder_tree1/12(din11)
  fir_tap11/4(imag) -> adder_tree2/12(din11)
  real12/1 -> fir_tap12/1(a)
  imag12/1 -> fir_tap12/2(b)
  fir_tap12/1(a_out) -> real_out12/1
  fir_tap12/2(b_out) -> imag_out12/1
  fir_tap12/3(real) -> adder_tree1/13(din12)
  fir_tap12/4(imag) -> adder_tree2/13(din12)
  real13/1 -> fir_tap13/1(a)
  imag13/1 -> fir_tap13/2(b)
  fir_tap13/1(a_out) -> real_out13/1
  fir_tap13/2(b_out) -> imag_out13/1
  fir_tap13/3(real) -> adder_tree1/14(din13)
  fir_tap13/4(imag) -> adder_tree2/14(din13)
  real14/1 -> fir_tap14/1(a)
  imag14/1 -> fir_tap14/2(b)
  fir_tap14/1(a_out) -> real_out14/1
  fir_tap14/2(b_out) -> imag_out14/1
  fir_tap14/3(real) -> adder_tree1/15(din14)
  fir_tap14/4(imag) -> adder_tree2/15(din14)
  real15/1 -> fir_tap15/1(a)
  imag15/1 -> fir_tap15/2(b)
  fir_tap15/1(a_out) -> real_out15/1
  fir_tap15/2(b_out) -> imag_out15/1
  fir_tap15/3(real) -> adder_tree1/16(din15)
  fir_tap15/4(imag) -> adder_tree2/16(din15)
  real16/1 -> fir_tap16/1(a)
  imag16/1 -> fir_tap16/2(b)
  fir_tap16/1(a_out) -> real_out16/1
  fir_tap16/2(b_out) -> imag_out16/1
  fir_tap16/3(real) -> adder_tree1/17(din16)
  fir_tap16/4(imag) -> adder_tree2/17(din16)
